simulink model "Closed_loop"  (R2023a)
settings: Solver=VariableStepAuto  StartTime=0.0  StopTime=500  RelTol=1e-3
values from neighbouring files (symbols this model uses):
  C_CLCS_D = charef_D(0.44)    [Final_Code.m]
  C_CLCS_I = charef_I(0.89)    [Final_Code.m]
libraries: cstblocks x5, fod x1
settings Model: Creator=xyz  LastModifiedBy=xyz

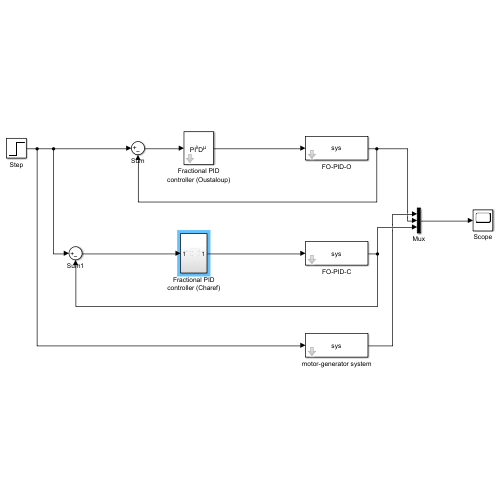
[thumbnail: Simulink's stored preview of the top-level diagram]
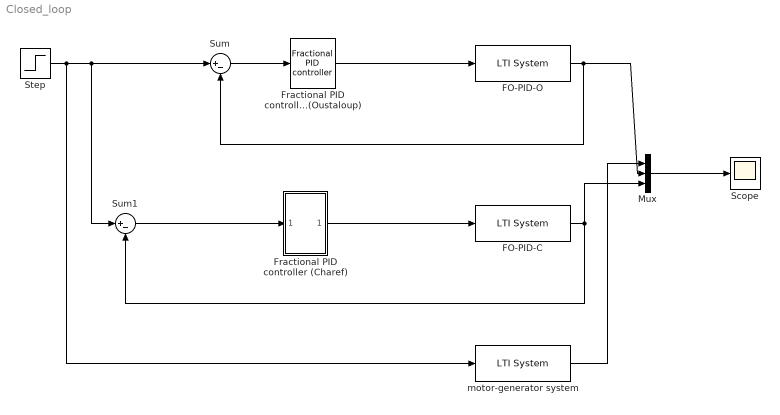
== system Closed_loop ==
  FO-PID-C : cstblocks/LTI System  sys=sys  IC=[]
  FO-PID-O : cstblocks/LTI System  sys=sys  IC=[]
  Fractional PID controller (Charef) : Subsystem
  Fractional PID controller (Oustaloup) : fod/Fractional PID controller  Kp=0.133  Ki=0.0532  lambda=0.89  Kd=0.10108  mic=0.44  freqRange=[0.001, 1000]  N=5
      settings: SourceProductName=FOMCON Toolbox
  Mux : Mux  Inputs=3
  Scope : Scope
  Step : Step  Time=0  SampleTime=0
  Sum : Sum  Inputs=|+-
  Sum1 : Sum  Inputs=|+-
  motor-generator system : cstblocks/LTI System  sys=sys  IC=[]
  wires:
  Step/1 -> motor-generator system/1, Sum/1, Sum1/1
  Sum/1 -> Fractional PID controller (Oustaloup)/1
  Fractional PID controller (Oustaloup)/1 -> FO-PID-O/1
  Mux/1 -> Scope/1
  FO-PID-O/1 -> Sum/2, Mux/2
  FO-PID-C/1 -> Mux/3, Sum1/2
  motor-generator system/1 -> Mux/1
  Sum1/1 -> Fractional PID controller (Charef)/1(In1)
  Fractional PID controller (Charef)/1(Out1) -> FO-PID-C/1

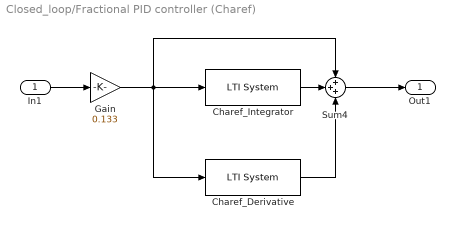
== system Closed_loop/Fractional PID controller (Charef) ==
  In1 : Inport
  Charef_Derivative : cstblocks/LTI System  sys=0.76*C_CLCS_D  IC=[]
  Charef_Integrator : cstblocks/LTI System  sys=(1/2.5)*C_CLCS_I  IC=[]
  Gain : Gain  Gain=0.133
  Sum4 : Sum  Inputs=+++
  Out1 : Outport
  wires:
  Charef_Derivative/1 -> Sum4/3
  Sum4/1 -> Out1/1
  Gain/1 -> Charef_Integrator/1, Sum4/1, Charef_Derivative/1
  Charef_Integrator/1 -> Sum4/2
  In1/1 -> Gain/1
